simulink model "eg242"  (R2014a)
settings: Solver=ode45  StartTime=0.0  StopTime=10.0  RelTol=1e-3
settings Model: Creator=tzb  LastModifiedBy=tzb

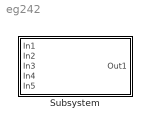
== system eg242 ==
  Subsystem : Subsystem  mask{Parameter1=[], Parameter2=0, Parameter3=<empty>, Parameter4=on, Parameter5=0}
      mask TypeOptions Parameter3: <empty>
      mask Display:
      | plot([0.2 0.4 0.6 0.8 0.2],[0.2 0.8 0.8 0.2 0.2])
      | disp('my function')

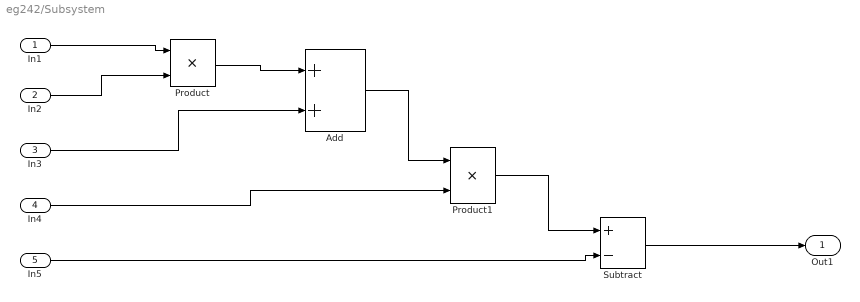
== system eg242/Subsystem ==
  In1 : Inport
  In2 : Inport  Port=2
  In3 : Inport  Port=3
  In4 : Inport  Port=4
  In5 : Inport  Port=5
  Add : Sum
  Product : Product
  Product1 : Product
  Subtract : Sum  Inputs=+-
  Out1 : Outport
  wires:
  In1/1 -> Product/1
  In2/1 -> Product/2
  Product/1 -> Add/1
  In3/1 -> Add/2
  Add/1 -> Product1/1
  In4/1 -> Product1/2
  Product1/1 -> Subtract/1
  In5/1 -> Subtract/2
  Subtract/1 -> Out1/1
